simulink model "IEEE39bus"  (Simulink 8.5)
settings: Solver=ode3  SolverMode=SingleTasking  StartTime=0.0  StopTime=50  FixedStep=Ts  RelTol=1e-3
PostLoadFcn:
  | Ts=25e-6; IEEE39BusLineLength;
  | vNomHV = 345E3;fNom=50;load('Dynamicload.mat');
InitFcn:
  | Ts=25e-6; IEEE39BusLineLength;
  | vNomHV = 345E3;fNom=50;load('Dynamicload.mat');
undefined symbols (not defined in the file): D1, Delta, load15, load16, load18, load20, load21, load23, load24, load25, load26, load27, load28, load29, load3, load39, load4, load7, load8, TL_10_11_len, TL_10_13_len, TL_13_14_len, TL_14_15_len, TL_15_16_len, TL_16_17_len, TL_16_19_len, TL_16_21_len, TL_16_24_len, TL_17_18_len, TL_17_27_len, TL_1_2_len, TL_1_39_len, TL_21_22_len, TL_22_23_len, TL_24_23_len, TL_25_26_len, TL_26_27_len, TL_26_28_len, TL_26_29_len, TL_28_29_len, TL_2_25_len, TL_2_2_len, TL_3_18_len, TL_3_4_len, TL_4_14_len, TL_4_5_len, TL_5_6_len, TL_5_8_len, TL_6_11_len, TL_6_7_len, TL_7_8_len, TL_8_9_len, TL_9_39_len
libraries: powerlib x175, op_dpl_lib x34, rtlab x14, sps_avr x9, powerlib_extras x2, artemis x1, powerlib_meascontrol x1
(part 2 of 5)

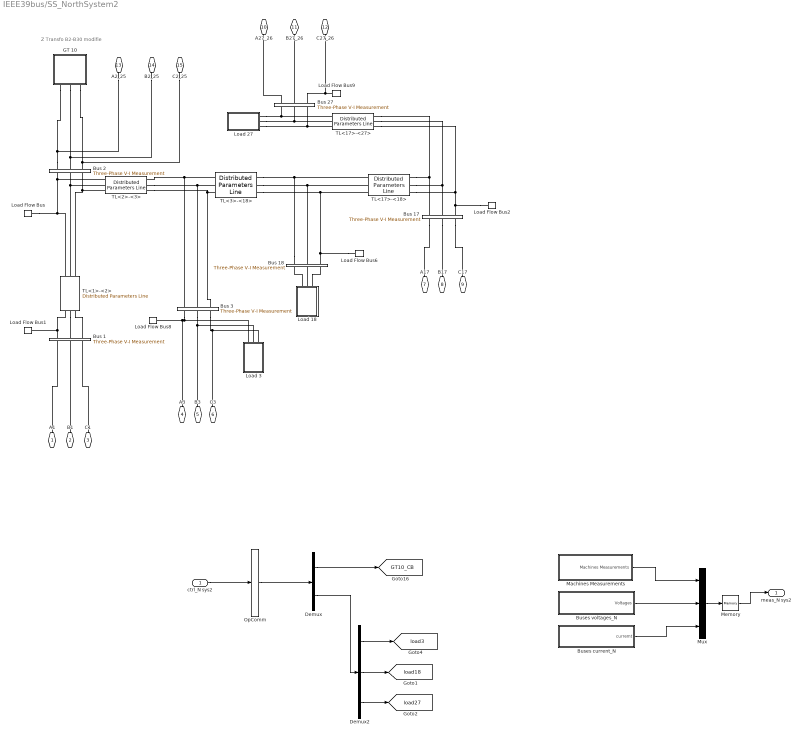
== system IEEE39bus/SS_NorthSystem2 ==
  note: Z Transfo B2-B30 modifie
  ctrl_N sys2 : Inport
  Bus 1 : powerlib/Measurements/Three-Phase V-I Measurement  VoltageMeasurement=phase-to-ground  SetLabelV=on  LabelV=V_bus_1  Vpu=off  VpuLL=off  CurrentMeasurement=yes  SetLabelI=on  LabelI=I_bus_1  Ipu=off  Pbase=100e6  Vbase=230e3  OutputType=Complex  PhasorSimulation=off  PSBequivalent=0
  Bus 17 : powerlib/Measurements/Three-Phase V-I Measurement  VoltageMeasurement=phase-to-ground  SetLabelV=on  LabelV=V_bus_17  Vpu=off  VpuLL=off  CurrentMeasurement=yes  SetLabelI=on  LabelI=I_bus_17  Ipu=off  Pbase=100e6  Vbase=230e3  OutputType=Complex  PhasorSimulation=off  PSBequivalent=0
  Bus 18 : powerlib/Measurements/Three-Phase V-I Measurement  VoltageMeasurement=phase-to-ground  SetLabelV=on  LabelV=V_bus_18  Vpu=off  VpuLL=off  CurrentMeasurement=yes  SetLabelI=on  LabelI=I_bus_18  Ipu=off  Pbase=100e6  Vbase=230e3  OutputType=Complex  PhasorSimulation=off  PSBequivalent=0
  Bus 2 : powerlib/Measurements/Three-Phase V-I Measurement  VoltageMeasurement=phase-to-ground  SetLabelV=on  LabelV=V_bus_2  Vpu=off  VpuLL=off  CurrentMeasurement=yes  SetLabelI=on  LabelI=I_bus_2  Ipu=off  Pbase=100e6  Vbase=230e3  OutputType=Complex  PhasorSimulation=off  PSBequivalent=0
  Bus 27 : powerlib/Measurements/Three-Phase V-I Measurement  VoltageMeasurement=phase-to-ground  SetLabelV=on  LabelV=V_bus_27  Vpu=off  VpuLL=off  CurrentMeasurement=yes  SetLabelI=on  LabelI=I_bus_27  Ipu=off  Pbase=100e6  Vbase=230e3  OutputType=Complex  PhasorSimulation=off  PSBequivalent=0
  Bus 3 : powerlib/Measurements/Three-Phase V-I Measurement  VoltageMeasurement=phase-to-ground  SetLabelV=on  LabelV=V_bus_3  Vpu=off  VpuLL=off  CurrentMeasurement=yes  SetLabelI=on  LabelI=I_bus_3  Ipu=off  Pbase=100e6  Vbase=230e3  OutputType=Complex  PhasorSimulation=off  PSBequivalent=0
  Buses current_N : Subsystem
  Buses voltages_N : Subsystem
  Demux : Demux  Outputs=[1 6]
  Demux2 : Demux  Outputs=[2 2 2]
  GT 10 : Subsystem
  Load 18 : Subsystem  SystemSampleTime=20e-3
  Load 27 : Subsystem  SystemSampleTime=20e-3
  Load 3 : Subsystem  SystemSampleTime=20e-3
  Load Flow Bus : powerlib/Measurements/Load Flow Bus  LConnTagsString=a  ID=Bus-2  Vbase=345e+003  Vref=1  Vangle=0  VLF=1.028  angleLF=24.05
      settings: AttributesFormatString=%<ID>\n%<Vbase>V\n%<VLF>pu\n%<angleLF>deg.
  Load Flow Bus1 : powerlib/Measurements/Load Flow Bus  LConnTagsString=a  ID=Bus-1  Vbase=345e+003  Vref=1  Vangle=0  VLF=1.036  angleLF=22.64
      settings: AttributesFormatString=%<ID>\n%<Vbase>V\n%<VLF>pu\n%<angleLF>deg.
  Load Flow Bus2 : powerlib/Measurements/Load Flow Bus  LConnTagsString=a  ID=Bus-17  Vbase=345e+003  Vref=1  Vangle=0  VLF=1.01  angleLF=19.53
      settings: AttributesFormatString=%<ID>\n%<Vbase>V\n%<VLF>pu\n%<angleLF>deg.
  Load Flow Bus6 : powerlib/Measurements/Load Flow Bus  LConnTagsString=a  ID=Bus-18  Vbase=345e+003  Vref=1  Vangle=0  VLF=1.009  angleLF=19.72
      settings: AttributesFormatString=%<ID>\n%<Vbase>V\n%<VLF>pu\n%<angleLF>deg.
  Load Flow Bus8 : powerlib/Measurements/Load Flow Bus  LConnTagsString=a  ID=Bus-3  Vbase=345e+003  Vref=1  Vangle=0  VLF=1.01  angleLF=21
      settings: AttributesFormatString=%<ID>\n%<Vbase>V\n%<VLF>pu\n%<angleLF>deg.
  Load Flow Bus9 : powerlib/Measurements/Load Flow Bus  LConnTagsString=a  ID=Bus-27  Vbase=345e+003  Vref=1  Vangle=0  VLF=1.013  angleLF=19.76
      settings: AttributesFormatString=%<ID>\n%<Vbase>V\n%<VLF>pu\n%<angleLF>deg.
  Machines Measurements : Subsystem
      mask Display: disp('Machines Measurements')
  Memory : Memory
  Mux : Mux  Inputs=3
  OpComm : rtlab/OpComm  nbport=1  groupe_acq=1  subsys_rate=0  st=0  Synchronization=on  Interpolation=on  Threshold=1.0  Missed_Data=off  Sim_Time=off  Samples=off  dynSigOut=off  from_console=0  warning_done=off  writeOpCommFile=off  Offset=off
  TL<17>-<18> : op_dpl_lib/Distributed Parameters Line  SimulationMode=ARTEMIS model  Phases=3  Frequency=50  Resistance=[0.833 3.333]/TL_17_18_len  Inductance="[0.026  0.078]/TL_17_18_len"  Capacitance=[0.294e-6 0.134e-6]/TL_17_18_len  Length=TL_17_18_len  Measurements=None
  TL<17>-<27> : op_dpl_lib/Distributed Parameters Line  SimulationMode=ARTEMIS model  Phases=3  Frequency=50  Resistance=[1.547 6.189]/TL_17_27_len  Inductance="[0.055  0.164]/TL_17_27_len"  Capacitance=[0.717e-6 0.326e-6]/TL_17_27_len  Length=TL_17_27_len  Measurements=None
  TL<1>-<2> : op_dpl_lib/Distributed Parameters Line  SimulationMode=ARTEMIS model  Phases=3  Frequency=50  Resistance=[4.166 16.66]/TL_1_2_len  Inductance="[0.13  0.389]/TL_1_2_len"  Capacitance=[1.56e-6 0.708e-6]/TL_1_2_len  Length=TL_1_2_len  Measurements=None
  TL<2>-<3> : op_dpl_lib/Distributed Parameters Line  SimulationMode=ARTEMIS model  Phases=3  Frequency=50  Resistance=[1.547 6.189]/TL_2_2_len  Inductance="[0.048  0.143]/TL_2_2_len"  Capacitance=[0.573e-6 0.261e-6]/TL_2_2_len  Length=TL_2_2_len  Measurements=None
  TL<3>-<18> : op_dpl_lib/Distributed Parameters Line  SimulationMode=ARTEMIS model  Phases=3  Frequency=50  Resistance=[1.309 5.237]/TL_3_18_len  Inductance="[0.042  0.126]/TL_3_18_len"  Capacitance=[0.476e-6 0.217e-6]/TL_3_18_len  Length=TL_3_18_len  Measurements=None
  A1 : PMIOPort  Port=1  Side=Left
  B1 : PMIOPort  Port=2  Side=Left
  C1 : PMIOPort  Port=3  Side=Left
  A3 : PMIOPort  Port=4  Side=Left
  B3 : PMIOPort  Port=5  Side=Left
  C3 : PMIOPort  Port=6  Side=Left
  A17 : PMIOPort  Port=7  Side=Left
  B17 : PMIOPort  Port=8  Side=Left
  C17 : PMIOPort  Port=9  Side=Left
  A27_26 : PMIOPort  Port=10  Side=Right
  B27_26 : PMIOPort  Port=11  Side=Right
  C27_26 : PMIOPort  Port=12  Side=Right
  A2_25 : PMIOPort  Port=13  Side=Right
  B2_25 : PMIOPort  Port=14  Side=Right
  C2_25 : PMIOPort  Port=15  Side=Right
  meas_N sys2 : Outport
  tag scope: GT10_CB=global, load18=global, load27=global, load3=global
  wires:
  Machines Measurements/1(Machines Measurements) -> Mux/1
  Mux/1 -> Memory/1
  Memory/1 -> meas_N sys2/1
  ctrl_N sys2/1 -> OpComm/1
  Buses voltages_N/1(Voltages) -> Mux/2
  Buses current_N/1(curremt) -> Mux/3
  Demux/2 -> Demux2/1
  Demux/1 -> [GT10_CB]
  Demux2/1 -> [load3]
  Demux2/3 -> [load27]
  Demux2/2 -> [load18]
  OpComm/1 -> Demux/1
  connections:
  TL<17>-<27>/LConn3 -- Load 27/LConn3 -- Bus 27/LConn3
  TL<17>-<27>/LConn2 -- Load 27/LConn2 -- Bus 27/LConn2
  TL<17>-<27>/LConn1 -- Load 27/LConn1 -- Bus 27/LConn1
  GT 10/RConn3 -- C2_25/RConn1 -- Bus 2/RConn3
  GT 10/RConn2 -- B2_25/RConn1 -- Bus 2/RConn2
  Bus 2/RConn1 -- GT 10/RConn1 -- A2_25/RConn1
  Load 18/LConn3 -- Bus 18/LConn3
  Load 18/LConn2 -- Bus 18/LConn2
  Load 18/LConn1 -- Bus 18/LConn1
  Load Flow Bus2/LConn1 -- TL<17>-<27>/RConn3 -- TL<17>-<18>/RConn3 -- Bus 17/RConn3
  TL<17>-<18>/RConn2 -- TL<17>-<27>/RConn2 -- Bus 17/RConn2
  TL<17>-<18>/RConn1 -- TL<17>-<27>/RConn1 -- Bus 17/RConn1
  TL<1>-<2>/RConn3 -- Bus 1/RConn3
  TL<1>-<2>/RConn2 -- Bus 1/RConn2
  Load Flow Bus1/LConn1 -- Bus 1/RConn1 -- TL<1>-<2>/RConn1
  TL<2>-<3>/LConn3 -- TL<1>-<2>/LConn3 -- Bus 2/LConn3
  TL<2>-<3>/LConn1 -- TL<1>-<2>/LConn1 -- Load Flow Bus/LConn1 -- Bus 2/LConn1
  TL<3>-<18>/LConn2 -- Bus 3/RConn2 -- TL<2>-<3>/RConn2
  TL<3>-<18>/LConn1 -- Bus 3/RConn1 -- TL<2>-<3>/RConn1
  TL<3>-<18>/LConn3 -- Bus 3/RConn3 -- TL<2>-<3>/RConn3
  Bus 3/LConn3 -- C3/RConn1 -- Load 3/LConn3
  Bus 3/LConn2 -- B3/RConn1 -- Load 3/LConn2
  Load Flow Bus8/LConn1 -- Load 3/LConn1 -- Bus 3/LConn1 -- A3/RConn1
  TL<2>-<3>/LConn2 -- TL<1>-<2>/LConn2 -- Bus 2/LConn2
  B1/RConn1 -- Bus 1/LConn2
  A1/RConn1 -- Bus 1/LConn1
  C1/RConn1 -- Bus 1/LConn3
  Bus 18/RConn1 -- TL<17>-<18>/LConn1 -- TL<3>-<18>/RConn1
  Bus 18/RConn2 -- TL<17>-<18>/LConn2 -- TL<3>-<18>/RConn2
  Load Flow Bus6/LConn1 -- TL<17>-<18>/LConn3 -- TL<3>-<18>/RConn3 -- Bus 18/RConn3
  Bus 17/LConn2 -- B17/RConn1
  Bus 17/LConn3 -- C17/RConn1
  Bus 17/LConn1 -- A17/RConn1
  Bus 27/RConn2 -- B27_26/RConn1
  Load Flow Bus9/LConn1 -- Bus 27/RConn3 -- C27_26/RConn1
  Bus 27/RConn1 -- A27_26/RConn1

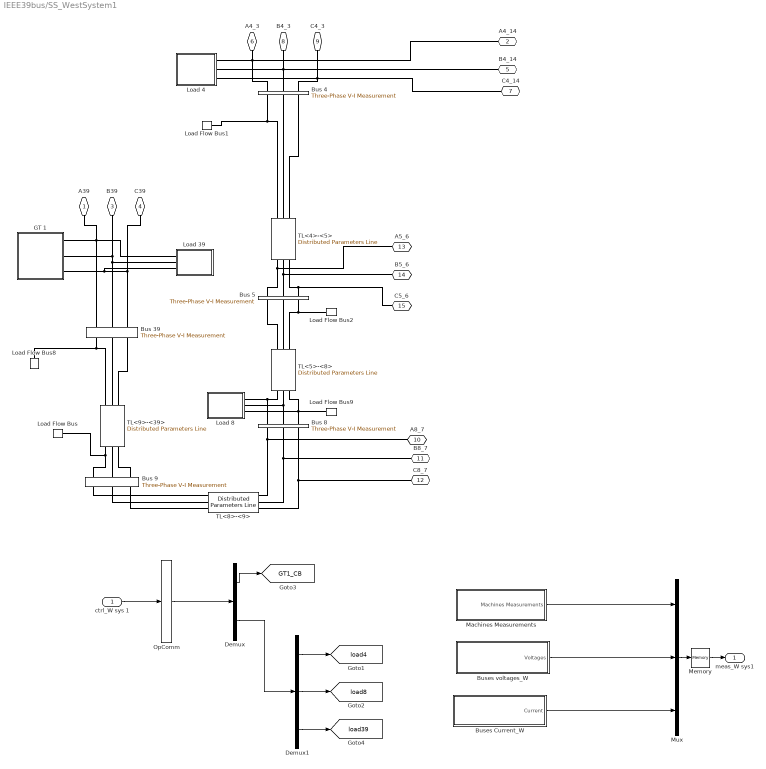
== system IEEE39bus/SS_WestSystem1 ==
  ctrl_W sys 1 : Inport
  Bus 39 : powerlib/Measurements/Three-Phase V-I Measurement  VoltageMeasurement=phase-to-ground  SetLabelV=on  LabelV=V_bus_39  Vpu=off  VpuLL=off  CurrentMeasurement=yes  SetLabelI=on  LabelI=I_bus_39  Ipu=off  Pbase=100e6  Vbase=345e3  OutputType=Complex  PhasorSimulation=off  PSBequivalent=0
  Bus 4 : powerlib/Measurements/Three-Phase V-I Measurement  VoltageMeasurement=phase-to-ground  SetLabelV=on  LabelV=V_bus_4  Vpu=off  VpuLL=off  CurrentMeasurement=yes  SetLabelI=on  LabelI=I_bus_4  Ipu=off  Pbase=100e6  Vbase=230e3  OutputType=Complex  PhasorSimulation=off  PSBequivalent=0
  Bus 5 : powerlib/Measurements/Three-Phase V-I Measurement  VoltageMeasurement=phase-to-ground  SetLabelV=on  LabelV=V_bus_5  Vpu=off  VpuLL=off  CurrentMeasurement=yes  SetLabelI=on  LabelI=I_bus_5  Ipu=off  Pbase=100e6  Vbase=230e3  OutputType=Complex  PhasorSimulation=off  PSBequivalent=0
  Bus 8 : powerlib/Measurements/Three-Phase V-I Measurement  VoltageMeasurement=phase-to-ground  SetLabelV=on  LabelV=V_bus_8  Vpu=off  VpuLL=off  CurrentMeasurement=yes  SetLabelI=on  LabelI=I_bus_8  Ipu=off  Pbase=100e6  Vbase=230e3  OutputType=Complex  PhasorSimulation=off  PSBequivalent=0
  Bus 9 : powerlib/Measurements/Three-Phase V-I Measurement  VoltageMeasurement=phase-to-ground  SetLabelV=on  LabelV=V_bus_9  Vpu=off  VpuLL=off  CurrentMeasurement=yes  SetLabelI=on  LabelI=I_bus_9  Ipu=off  Pbase=100e6  Vbase=230e3  OutputType=Complex  PhasorSimulation=off  PSBequivalent=0
  Buses Current_W : Subsystem
  Buses voltages_W : Subsystem
  Demux : Demux  Outputs=[1 6]
  Demux1 : Demux  Outputs=[2 2 2]
  "GT 1 " : Subsystem
  Load 39 : Subsystem  SystemSampleTime=20e-3
  Load 4 : Subsystem
  Load 8 : Subsystem
  Load Flow Bus : powerlib/Measurements/Load Flow Bus  LConnTagsString=a  ID=Bus-9  Vbase=345e+003  Vref=1  Vangle=0  VLF=1.022  angleLF=20.59
      settings: AttributesFormatString=%<ID>\n%<Vbase>V\n%<VLF>pu\n%<angleLF>deg.
  Load Flow Bus1 : powerlib/Measurements/Load Flow Bus  LConnTagsString=a  ID=Bus-4  Vbase=345e+003  Vref=1  Vangle=0  VLF=0.9935  angleLF=19.16
      settings: AttributesFormatString=%<ID>\n%<Vbase>V\n%<VLF>pu\n%<angleLF>deg.
  Load Flow Bus2 : powerlib/Measurements/Load Flow Bus  LConnTagsString=a  ID=Bus-5  Vbase=345e+003  Vref=1  Vangle=0  VLF=0.9982  angleLF=20.09
      settings: AttributesFormatString=%<ID>\n%<Vbase>V\n%<VLF>pu\n%<angleLF>deg.
  Load Flow Bus8 : powerlib/Measurements/Load Flow Bus  LConnTagsString=a  ID=Bus-39  Vbase=345000  Vref=1.03  Vangle=0  VLF=1.029  angleLF=21.84
      settings: AttributesFormatString=%<ID>\n%<Vbase>V\n%<VLF>pu\n%<angleLF>deg.
  Load Flow Bus9 : powerlib/Measurements/Load Flow Bus  LConnTagsString=a  ID=Bus-8  Vbase=345e+003  Vref=1  Vangle=0  VLF=0.9916  angleLF=18.81
      settings: AttributesFormatString=%<ID>\n%<Vbase>V\n%<VLF>pu\n%<angleLF>deg.
  Machines Measurements : Subsystem
      mask Display: disp('Machines Measurements')
  Memory : Memory
  Mux : Mux  Inputs=3
  OpComm : rtlab/OpComm  nbport=1  groupe_acq=1  subsys_rate=0  st=0  Synchronization=on  Interpolation=on  Threshold=1.0  Missed_Data=off  Sim_Time=off  Samples=off  dynSigOut=off  from_console=0  warning_done=off  writeOpCommFile=off  Offset=off
  TL<4>-<5> : op_dpl_lib/Distributed Parameters Line  SimulationMode=ARTEMIS model  Phases=3  Frequency=50  Resistance=[0.952 3.809]/TL_4_5_len  Inductance="[0.04  0.121]/TL_4_5_len"  Capacitance=[0.299e-6 0.136e-6]/TL_4_5_len  Length=TL_4_5_len  Measurements=None
  TL<5>-<8> : op_dpl_lib/Distributed Parameters Line  SimulationMode=ARTEMIS model  Phases=3  Frequency=50  Resistance=[0.952 3.809]/TL_5_8_len  Inductance="[0.035  0.106]/TL_5_8_len"  Capacitance=[0.329e-6 0.15e-6]/TL_5_8_len  Length=TL_5_8_len  Measurements=None
  TL<8>-<9> : op_dpl_lib/Distributed Parameters Line  SimulationMode=ARTEMIS model  Phases=3  Frequency=50  Resistance=[2.738 10.95]/TL_8_9_len  Inductance="[0.115  0.344]/TL_8_9_len"  Capacitance=[0.848e-6 0.385e-6]/TL_8_9_len  Length=TL_8_9_len  Measurements=None
  TL<9>-<39> : op_dpl_lib/Distributed Parameters Line  SimulationMode=ARTEMIS model  Phases=3  Frequency=50  Resistance=[1.19 4.761]/TL_9_39_len  Inductance="[0.079  0.237]/TL_9_39_len"  Capacitance=[2.674e-6 1.216e-6]/TL_9_39_len  Length=TL_9_39_len  Measurements=None
  A39 : PMIOPort  Port=1  Side=Right
  A4_14 : PMIOPort  Port=2  Side=Left
  B39 : PMIOPort  Port=3  Side=Right
  C39 : PMIOPort  Port=4  Side=Right
  B4_14 : PMIOPort  Port=5  Side=Left
  A4_3 : PMIOPort  Port=6  Side=Right
  C4_14 : PMIOPort  Port=7  Side=Left
  B4_3 : PMIOPort  Port=8  Side=Right
  C4_3 : PMIOPort  Port=9  Side=Right
  A8_7 : PMIOPort  Port=10  Side=Left
  B8_7 : PMIOPort  Port=11  Side=Left
  C8_7 : PMIOPort  Port=12  Side=Left
  A5_6 : PMIOPort  Port=13  Side=Right
  B5_6 : PMIOPort  Port=14  Side=Right
  C5_6 : PMIOPort  Port=15  Side=Right
  meas_W sys1 : Outport
  tag scope: GT1_CB=global, load39=global, load4=global, load8=global
  wires:
  ctrl_W sys 1/1 -> OpComm/1
  OpComm/1 -> Demux/1
  Mux/1 -> Memory/1
  Memory/1 -> meas_W sys1/1
  Buses voltages_W/1(Voltages) -> Mux/2
  Machines Measurements/1(Machines Measurements) -> Mux/1
  Buses Current_W/1(Current) -> Mux/3
  Demux/1 -> [GT1_CB]
  Demux/2 -> Demux1/1
  Demux1/2 -> [load8]
  Demux1/1 -> [load4]
  Demux1/3 -> [load39]
  connections:
  Bus 9/RConn3 -- TL<9>-<39>/RConn3
  Bus 9/RConn2 -- TL<9>-<39>/RConn2
  Bus 9/RConn1 -- Load Flow Bus/LConn1 -- TL<9>-<39>/RConn1
  Load Flow Bus9/LConn1 -- Load 8/LConn3 -- TL<5>-<8>/RConn3 -- Bus 8/RConn3
  TL<5>-<8>/RConn2 -- Load 8/LConn2 -- Bus 8/RConn2
  TL<5>-<8>/RConn1 -- Load 8/LConn1 -- Bus 8/RConn1
  TL<8>-<9>/RConn3 -- Bus 8/LConn3 -- C8_7/RConn1
  TL<8>-<9>/RConn2 -- Bus 8/LConn2 -- B8_7/RConn1
  TL<8>-<9>/RConn1 -- A8_7/RConn1 -- Bus 8/LConn1
  Bus 5/RConn3 -- TL<4>-<5>/RConn3 -- C5_6/RConn1
  Bus 5/RConn2 -- B5_6/RConn1 -- TL<4>-<5>/RConn2
  Bus 5/RConn1 -- A5_6/RConn1 -- TL<4>-<5>/RConn1
  "GT 1 "/RConn3 -- Bus 39/RConn3 -- C39/RConn1 -- Load 39/LConn3
  "GT 1 "/RConn2 -- Load 39/LConn2 -- Bus 39/RConn2 -- B39/RConn1
  Bus 39/RConn1 -- Load 39/LConn1 -- "GT 1 "/RConn1 -- A39/RConn1
  Load Flow Bus8/LConn1 -- TL<9>-<39>/LConn1 -- Bus 39/LConn1
  Bus 39/LConn2 -- TL<9>-<39>/LConn2
  Bus 39/LConn3 -- TL<9>-<39>/LConn3
  Bus 9/LConn1 -- TL<8>-<9>/LConn1
  Bus 9/LConn2 -- TL<8>-<9>/LConn2
  Bus 9/LConn3 -- TL<8>-<9>/LConn3
  Bus 5/LConn1 -- TL<5>-<8>/LConn1
  Bus 5/LConn2 -- TL<5>-<8>/LConn2
  Load Flow Bus2/LConn1 -- TL<5>-<8>/LConn3 -- Bus 5/LConn3
  Load Flow Bus1/LConn1 -- TL<4>-<5>/LConn1 -- Bus 4/LConn1
  Bus 4/LConn2 -- TL<4>-<5>/LConn2
  Bus 4/LConn3 -- TL<4>-<5>/LConn3
  B4_3/RConn1 -- B4_14/RConn1 -- Load 4/LConn2 -- Bus 4/RConn2
  A4_3/RConn1 -- A4_14/RConn1 -- Load 4/LConn1 -- Bus 4/RConn1
  C4_3/RConn1 -- C4_14/RConn1 -- Load 4/LConn3 -- Bus 4/RConn3

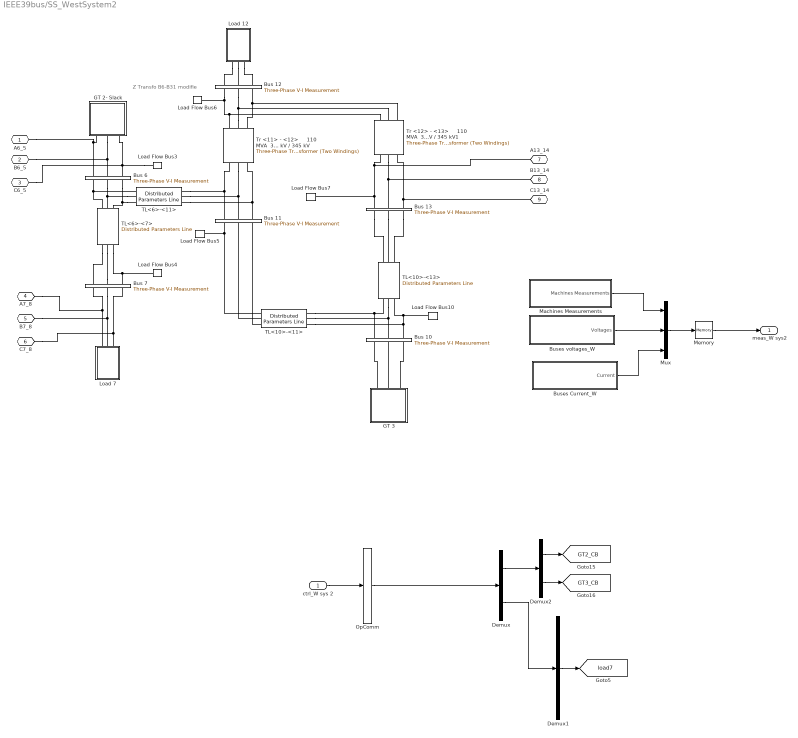
== system IEEE39bus/SS_WestSystem2 ==
  note: Z Transfo B6-B31 modifie
  ctrl_W sys 2 : Inport
  Bus 10 : powerlib/Measurements/Three-Phase V-I Measurement  VoltageMeasurement=phase-to-ground  SetLabelV=on  LabelV=V_bus_10  Vpu=off  VpuLL=off  CurrentMeasurement=yes  SetLabelI=on  LabelI=I_bus_10  Ipu=off  Pbase=100e6  Vbase=230e3  OutputType=Complex  PhasorSimulation=off  PSBequivalent=0
  Bus 11 : powerlib/Measurements/Three-Phase V-I Measurement  VoltageMeasurement=phase-to-ground  SetLabelV=on  LabelV=V_bus_11  Vpu=off  VpuLL=off  CurrentMeasurement=yes  SetLabelI=on  LabelI=I_bus_11  Ipu=off  Pbase=100e6  Vbase=230e3  OutputType=Complex  PhasorSimulation=off  PSBequivalent=0
  Bus 12 : powerlib/Measurements/Three-Phase V-I Measurement  VoltageMeasurement=phase-to-ground  SetLabelV=on  LabelV=V_bus_12  Vpu=off  VpuLL=off  CurrentMeasurement=yes  SetLabelI=on  LabelI=I_bus_12  Ipu=off  Pbase=100e6  Vbase=230e3  OutputType=Complex  PhasorSimulation=off  PSBequivalent=0
  Bus 13 : powerlib/Measurements/Three-Phase V-I Measurement  VoltageMeasurement=phase-to-ground  SetLabelV=on  LabelV=V_bus_13  Vpu=off  VpuLL=off  CurrentMeasurement=yes  SetLabelI=on  LabelI=I_bus_13  Ipu=off  Pbase=100e6  Vbase=230e3  OutputType=Complex  PhasorSimulation=off  PSBequivalent=0
  Bus 6 : powerlib/Measurements/Three-Phase V-I Measurement  VoltageMeasurement=phase-to-ground  SetLabelV=on  LabelV=V_bus_6  Vpu=off  VpuLL=off  CurrentMeasurement=yes  SetLabelI=on  LabelI=I_bus_6  Ipu=off  Pbase=100e6  Vbase=230e3  OutputType=Complex  PhasorSimulation=off  PSBequivalent=0
  Bus 7 : powerlib/Measurements/Three-Phase V-I Measurement  VoltageMeasurement=phase-to-ground  SetLabelV=on  LabelV=V_bus_7  Vpu=off  VpuLL=off  CurrentMeasurement=yes  SetLabelI=on  LabelI=I_bus_7  Ipu=off  Pbase=100e6  Vbase=230e3  OutputType=Complex  PhasorSimulation=off  PSBequivalent=0
  Buses Current_W : Subsystem
  Buses voltages_W : Subsystem
  Demux : Demux  Outputs=[2 2]
  Demux1 : Demux  Outputs=[2 ]
  Demux2 : Demux  Outputs=2
  GT 2- Slack : Subsystem
  GT 3 : Subsystem
  Load 12 : Subsystem
  Load 7 : Subsystem
  Load Flow Bus10 : powerlib/Measurements/Load Flow Bus  LConnTagsString=a  ID=Bus-10  Vbase=345e+003  Vref=1  Vangle=0  VLF=1.011  angleLF=22.22
      settings: AttributesFormatString=%<ID>\n%<Vbase>V\n%<VLF>pu\n%<angleLF>deg.
  Load Flow Bus3 : powerlib/Measurements/Load Flow Bus  LConnTagsString=a  ID=Bus-6  Vbase=345e+003  Vref=1  Vangle=0  VLF=1.003  angleLF=20.92
      settings: AttributesFormatString=%<ID>\n%<Vbase>V\n%<VLF>pu\n%<angleLF>deg.
  Load Flow Bus4 : powerlib/Measurements/Load Flow Bus  LConnTagsString=a  ID=Bus-7  Vbase=345e+003  Vref=1  Vangle=0  VLF=0.9928  angleLF=19.19
      settings: AttributesFormatString=%<ID>\n%<Vbase>V\n%<VLF>pu\n%<angleLF>deg.
  Load Flow Bus5 : powerlib/Measurements/Load Flow Bus  LConnTagsString=a  ID=Bus-11  Vbase=345e+003  Vref=1  Vangle=0  VLF=1.007  angleLF=21.76
      settings: AttributesFormatString=%<ID>\n%<Vbase>V\n%<VLF>pu\n%<angleLF>deg.
  Load Flow Bus6 : powerlib/Measurements/Load Flow Bus  LConnTagsString=a  ID=Bus-12  Vbase=345e+003  Vref=1  Vangle=0  VLF=0.996  angleLF=51.6
      settings: AttributesFormatString=%<ID>\n%<Vbase>V\n%<VLF>pu\n%<angleLF>deg.
  Load Flow Bus7 : powerlib/Measurements/Load Flow Bus  LConnTagsString=a  ID=Bus-13  Vbase=345e+003  Vref=1  Vangle=0  VLF=1.007  angleLF=21.59
      settings: AttributesFormatString=%<ID>\n%<Vbase>V\n%<VLF>pu\n%<angleLF>deg.
  Machines Measurements : Subsystem
      mask Display: disp('Machines Measurements')
  Memory : Memory
  Mux : Mux  Inputs=3
  OpComm : rtlab/OpComm  nbport=1  groupe_acq=1  subsys_rate=0  st=0  Synchronization=on  Interpolation=on  Threshold=1.0  Missed_Data=off  Sim_Time=off  Samples=off  dynSigOut=off  from_console=0  warning_done=off  writeOpCommFile=off  Offset=off
  TL<10>-<11> : op_dpl_lib/Distributed Parameters Line  SimulationMode=ARTEMIS model  Phases=3  Frequency=50  Resistance=[0.476 1.904]/TL_10_11_len  Inductance="[0.014  0.04]/TL_10_11_len"  Capacitance=[0.162e-6 0.074e-6]/TL_10_11_len  Length=TL_10_11_len  Measurements=None
  TL<10>-<13> : op_dpl_lib/Distributed Parameters Line  SimulationMode=ARTEMIS model  Phases=3  Frequency=50  Resistance=[0.476 1.904]/TL_10_13_len  Inductance="[0.014  0.04]/TL_10_13_len"  Capacitance=[0.162e-6 0.074e-6]/TL_10_13_len  Length=TL_10_13_len  Measurements=None
  TL<6>-<11> : op_dpl_lib/Distributed Parameters Line  SimulationMode=ARTEMIS model  Phases=3  Frequency=50  Resistance=[0.833 3.333]/TL_6_11_len  Inductance="[0.026  0.078]/TL_6_11_len"  Capacitance=[0.31e-6 0.141e-6]/TL_6_11_len  Length=TL_6_11_len  Measurements=None
  TL<6>-<7> : op_dpl_lib/Distributed Parameters Line  SimulationMode=ARTEMIS model  Phases=3  Frequency=50  Resistance=[0.714 2.857]/TL_6_7_len  Inductance="[0.029  0.087]/TL_6_7_len"  Capacitance=[0.252e-6 0.114e-6]/TL_6_7_len  Length=TL_6_7_len  Measurements=None
  Tr <11> - <12>     110 MVA  345 kV / 345 kV : powerlib/Elements/Three-Phase Transformer (Two Windings)  Winding1Connection=Delta (D1)  Winding2Connection=Yg  CoreType=Three single-phase transformers  SetSaturation=off  Hysteresis=off  DataFile='hysteresis'  SetInitialFlux=off  Measurements=None  UNITS=pu  NominalPower=[ 110e6 50]  Winding1="[345e3 0.0016*110/100/2   0.0435*110/100/2]"  Winding2="[ 1.006*345e3 0.0016*110/100/2   0.0435*110/100/2]"  Rm=500  Lm=500  L0=0.5  Saturation="[ 0,0  ;  0.005,1.2  ;  1.0,1.4 ]"  InitialFluxes=[ 0.8 , -0.8 , 0.7 ]  MoreParameters=off  BreakLoop=off  DataType=off  TransfoNumber=0
  Tr <12> - <13>     110 MVA  345 kV / 345 kV1 : powerlib/Elements/Three-Phase Transformer (Two Windings)  Winding1Connection=Delta (D1)  Winding2Connection=Yg  CoreType=Three single-phase transformers  SetSaturation=off  Hysteresis=off  DataFile='hysteresis'  SetInitialFlux=off  Measurements=None  UNITS=pu  NominalPower=[ 110e6 50]  Winding1="[ 345e3  0.0016*110/100/2   0.0435*110/100/2]"  Winding2="[ 1.006*345e3  0.0016*110/100/2   0.0435*110/100/2]"  Rm=500  Lm=500  L0=0.5  Saturation="[ 0,0  ;  0.005,1.2  ;  1.0,1.4 ]"  InitialFluxes=[ 0.8 , -0.8 , 0.7 ]  MoreParameters=off  BreakLoop=off  DataType=off  TransfoNumber=0
  A6_5 : PMIOPort  Port=1  Side=Left
  B6_5 : PMIOPort  Port=2  Side=Left
  C6_5 : PMIOPort  Port=3  Side=Left
  A7_8 : PMIOPort  Port=4  Side=Left
  B7_8 : PMIOPort  Port=5  Side=Left
  C7_8 : PMIOPort  Port=6  Side=Left
  A13_14 : PMIOPort  Port=7  Side=Right
  B13_14 : PMIOPort  Port=8  Side=Right
  C13_14 : PMIOPort  Port=9  Side=Right
  meas_W sys2 : Outport
  tag scope: GT2_CB=global, GT3_CB=global, load7=global
  wires:
  Mux/1 -> Memory/1
  Memory/1 -> meas_W sys2/1
  Buses voltages_W/1(Voltages) -> Mux/2
  Machines Measurements/1(Machines Measurements) -> Mux/1
  Buses Current_W/1(Current) -> Mux/3
  ctrl_W sys 2/1 -> OpComm/1
  OpComm/1 -> Demux/1
  Demux/2 -> Demux1/1
  Demux/1 -> Demux2/1
  Demux2/1 -> [GT2_CB]
  Demux2/2 -> [GT3_CB]
  Demux1/1 -> [load7]
  connections:
  Bus 7/RConn3 -- TL<6>-<7>/RConn3 -- Load Flow Bus4/LConn1
  Load Flow Bus3/LConn1 -- C6_5/RConn1 -- GT 2- Slack/RConn3 -- Bus 6/RConn3
  GT 2- Slack/RConn2 -- B6_5/RConn1 -- Bus 6/RConn2
  GT 2- Slack/RConn1 -- Bus 6/RConn1 -- A6_5/RConn1
  TL<6>-<11>/LConn3 -- TL<6>-<7>/LConn3 -- Bus 6/LConn3
  TL<6>-<11>/LConn2 -- TL<6>-<7>/LConn2 -- Bus 6/LConn2
  TL<6>-<7>/LConn1 -- Bus 6/LConn1 -- TL<6>-<11>/LConn1
  Bus 13/RConn3 -- Tr <12> - <13>     110 MVA  345 kV / 345 kV1/LConn3 -- C13_14/RConn1
  Tr <12> - <13>     110 MVA  345 kV / 345 kV1/LConn2 -- Bus 13/RConn2 -- B13_14/RConn1
  Load Flow Bus7/LConn1 -- Bus 13/RConn1 -- Tr <12> - <13>     110 MVA  345 kV / 345 kV1/LConn1 -- A13_14/RConn1
  Load 12/LConn3 -- Bus 12/RConn3
  Load 12/LConn2 -- Bus 12/RConn2
  Load 12/LConn1 -- Bus 12/RConn1
  Bus 12/LConn3 -- Tr <11> - <12>     110 MVA  345 kV / 345 kV/RConn3 -- Tr <12> - <13>     110 MVA  345 kV / 345 kV1/RConn3
  Tr <11> - <12>     110 MVA  345 kV / 345 kV/RConn2 -- Bus 12/LConn2 -- Tr <12> - <13>     110 MVA  345 kV / 345 kV1/RConn2
  Load Flow Bus6/LConn1 -- Tr <12> - <13>     110 MVA  345 kV / 345 kV1/RConn1 -- Tr <11> - <12>     110 MVA  345 kV / 345 kV/RConn1 -- Bus 12/LConn1
  Bus 11/RConn3 -- TL<6>-<11>/RConn3 -- Tr <11> - <12>     110 MVA  345 kV / 345 kV/LConn3
  Tr <11> - <12>     110 MVA  345 kV / 345 kV/LConn2 -- TL<6>-<11>/RConn2 -- Bus 11/RConn2
  Tr <11> - <12>     110 MVA  345 kV / 345 kV/LConn1 -- TL<6>-<11>/RConn1 -- Bus 11/RConn1
  TL<10>-<11>/LConn3 -- Bus 11/LConn3
  TL<10>-<11>/LConn2 -- Bus 11/LConn2
  Load Flow Bus5/LConn1 -- TL<10>-<11>/LConn1 -- Bus 11/LConn1
  TL<10>-<13>/RConn3 -- TL<10>-<11>/RConn3 -- Bus 10/RConn3 -- Load Flow Bus10/LConn1
  TL<10>-<13>/RConn2 -- TL<10>-<11>/RConn2 -- Bus 10/RConn2
  Bus 10/RConn1 -- TL<10>-<11>/RConn1 -- TL<10>-<13>/RConn1
  GT 3/RConn3 -- Bus 10/LConn3
  GT 3/RConn2 -- Bus 10/LConn2
  GT 3/RConn1 -- Bus 10/LConn1
  Bus 7/LConn1 -- A7_8/RConn1 -- Load 7/LConn1
  Bus 7/LConn2 -- Load 7/LConn2 -- B7_8/RConn1
  Bus 7/LConn3 -- C7_8/RConn1 -- Load 7/LConn3
  TL<6>-<7>/RConn2 -- Bus 7/RConn2
  TL<6>-<7>/RConn1 -- Bus 7/RConn1
  Bus 13/LConn1 -- TL<10>-<13>/LConn1
  Bus 13/LConn2 -- TL<10>-<13>/LConn2
  Bus 13/LConn3 -- TL<10>-<13>/LConn3

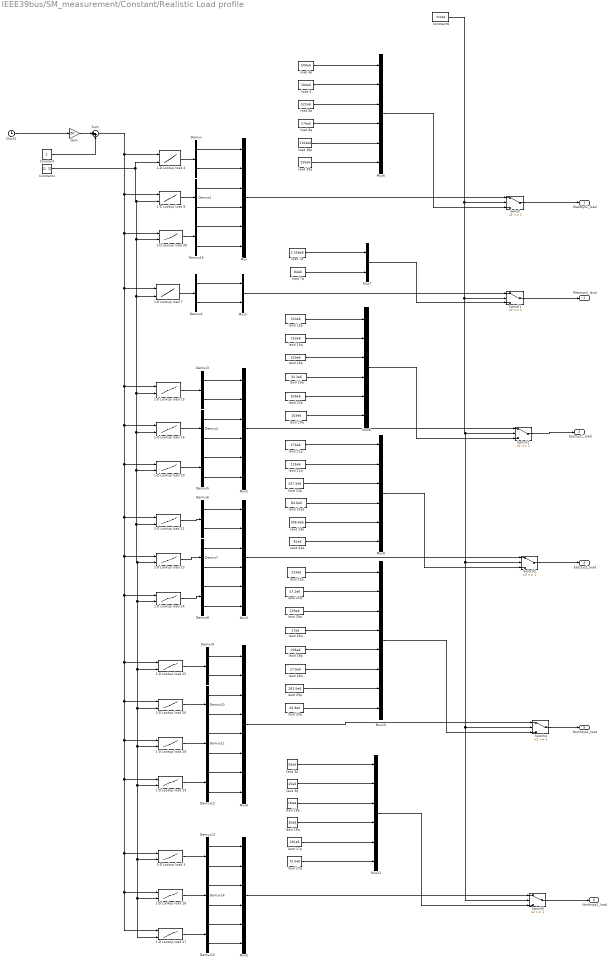
== system IEEE39bus/SM_measurement/Constant/Realistic Load profile ==
  1-D Lookup load 15 : Lookup_n-D  BreakpointsForDimension1=[1:18000]  BreakpointsForDimension2=[1 2]  Table=load15  InterpMethod=Flat  ExtrapMethod=Cubic spline  DiagnosticForOutOfRangeInput=Error  InternalRulePriority=Speed  RndMeth=Simplest  InputSameDT=on
  1-D Lookup load 16 : Lookup_n-D  BreakpointsForDimension1=[1:18000]  BreakpointsForDimension2=[1 2]  Table=load16  InterpMethod=Flat  ExtrapMethod=Cubic spline  DiagnosticForOutOfRangeInput=Error  InternalRulePriority=Speed  RndMeth=Simplest  InputSameDT=on
  1-D Lookup load 18 : Lookup_n-D  BreakpointsForDimension1=[1:18000]  BreakpointsForDimension2=[1 2]  Table=load18  InterpMethod=Flat  ExtrapMethod=Cubic spline  DiagnosticForOutOfRangeInput=Error  InternalRulePriority=Speed  RndMeth=Simplest  InputSameDT=on
  1-D Lookup load 20 : Lookup_n-D  BreakpointsForDimension1=[1:18000]  BreakpointsForDimension2=[1 2]  Table=load20  InterpMethod=Flat  ExtrapMethod=Cubic spline  DiagnosticForOutOfRangeInput=Error  InternalRulePriority=Speed  RndMeth=Simplest  InputSameDT=on
  1-D Lookup load 21 : Lookup_n-D  BreakpointsForDimension1=[1:18000]  BreakpointsForDimension2=[1 2]  Table=load21  InterpMethod=Flat  ExtrapMethod=Cubic spline  DiagnosticForOutOfRangeInput=Error  InternalRulePriority=Speed  RndMeth=Simplest  InputSameDT=on
  1-D Lookup load 23 : Lookup_n-D  BreakpointsForDimension1=[1:18000]  BreakpointsForDimension2=[1 2]  Table=load23  InterpMethod=Flat  ExtrapMethod=Cubic spline  DiagnosticForOutOfRangeInput=Error  InternalRulePriority=Speed  RndMeth=Simplest  InputSameDT=on
  1-D Lookup load 24 : Lookup_n-D  BreakpointsForDimension1=[1:18000]  BreakpointsForDimension2=[1 2]  Table=load24  InterpMethod=Flat  ExtrapMethod=Cubic spline  DiagnosticForOutOfRangeInput=Error  InternalRulePriority=Speed  RndMeth=Simplest  InputSameDT=on
  1-D Lookup load 25 : Lookup_n-D  BreakpointsForDimension1=[1:18000]  BreakpointsForDimension2=[1 2]  Table=load25  InterpMethod=Flat  ExtrapMethod=Cubic spline  DiagnosticForOutOfRangeInput=Error  InternalRulePriority=Speed  RndMeth=Simplest  InputSameDT=on
  1-D Lookup load 26 : Lookup_n-D  BreakpointsForDimension1=[1:18000]  BreakpointsForDimension2=[1 2]  Table=load26  InterpMethod=Flat  ExtrapMethod=Cubic spline  DiagnosticForOutOfRangeInput=Error  InternalRulePriority=Speed  RndMeth=Simplest  InputSameDT=on
  1-D Lookup load 27 : Lookup_n-D  BreakpointsForDimension1=[1:18000]  BreakpointsForDimension2=[1 2]  Table=load27  InterpMethod=Flat  ExtrapMethod=Cubic spline  DiagnosticForOutOfRangeInput=Error  InternalRulePriority=Speed  RndMeth=Simplest  InputSameDT=on
  1-D Lookup load 28 : Lookup_n-D  BreakpointsForDimension1=[1:18000]  BreakpointsForDimension2=[1 2]  Table=load28  InterpMethod=Flat  ExtrapMethod=Cubic spline  DiagnosticForOutOfRangeInput=Error  InternalRulePriority=Speed  RndMeth=Simplest  InputSameDT=on
  1-D Lookup load 29 : Lookup_n-D  BreakpointsForDimension1=[1:18000]  BreakpointsForDimension2=[1 2]  Table=load29  InterpMethod=Flat  ExtrapMethod=Cubic spline  DiagnosticForOutOfRangeInput=Error  InternalRulePriority=Speed  RndMeth=Simplest  InputSameDT=on
  1-D Lookup load 3 : Lookup_n-D  BreakpointsForDimension1=[1:18000]  BreakpointsForDimension2=[1 2]  Table=load3  InterpMethod=Flat  ExtrapMethod=Cubic spline  DiagnosticForOutOfRangeInput=Error  InternalRulePriority=Speed  RndMeth=Simplest  InputSameDT=on
  1-D Lookup load 39 : Lookup_n-D  BreakpointsForDimension1=[1:18000]  BreakpointsForDimension2=[1 2]  Table=load39  InterpMethod=Flat  ExtrapMethod=Cubic spline  DiagnosticForOutOfRangeInput=Error  InternalRulePriority=Speed  RndMeth=Simplest  InputSameDT=on
  1-D Lookup load 4 : Lookup_n-D  BreakpointsForDimension1=[1:18000]  BreakpointsForDimension2=[1 2]  Table=load4  InterpMethod=Flat  ExtrapMethod=Cubic spline  DiagnosticForOutOfRangeInput=Error  InternalRulePriority=Speed  RndMeth=Simplest  InputSameDT=on
  1-D Lookup load 7 : Lookup_n-D  BreakpointsForDimension1=[1:18000]  BreakpointsForDimension2=[1 2]  Table=load7  InterpMethod=Flat  ExtrapMethod=Cubic spline  DiagnosticForOutOfRangeInput=Error  InternalRulePriority=Speed  RndMeth=Simplest  InputSameDT=on
  1-D Lookup load 8 : Lookup_n-D  BreakpointsForDimension1=[1:18000]  BreakpointsForDimension2=[1 2]  Table=load8  InterpMethod=Flat  ExtrapMethod=Cubic spline  DiagnosticForOutOfRangeInput=Error  InternalRulePriority=Speed  RndMeth=Simplest  InputSameDT=on
  Clock1 : Clock
  Constant : Constant  SampleTime=20e-3
  Constant1 : Constant  Value="[1  2]"  VectorParams1D=off  SampleTime=20e-3
  Constant6 : Constant  Value=mode
  Demux{,1..16} (17 alike) : Demux  Outputs=2
  Gain : Gain  Gain=50
  Mux{,2..3,5..6,8..9,11} (8 alike) : Mux  Inputs=6
  Mux1 : Mux  Inputs=2
  Mux10 : Mux  Inputs=8
  Mux4 : Mux  Inputs=8
  Mux7 : Mux  Inputs=2
  Sum : Sum  Inputs=|++
  Switch{,1..5} (6 alike) : Switch  Threshold=1
  laod 15p : Constant  Value=320e6  VectorParams1D=off  SampleTime=20e-3
  laod 15q : Constant  Value=153e6  VectorParams1D=off  SampleTime=20e-3
  laod 16p : Constant  Value=329e6  VectorParams1D=off  SampleTime=20e-3
  laod 16q : Constant  Value=32.3e6  VectorParams1D=off  SampleTime=20e-3
  laod 18p : Constant  Value=158e6  VectorParams1D=off  SampleTime=20e-3
  laod 18q : Constant  Value=30e6  VectorParams1D=off  SampleTime=20e-3
  laod 20p : Constant  Value=628e6  VectorParams1D=off  SampleTime=20e-3
  laod 20q : Constant  Value=103e6  VectorParams1D=off  SampleTime=20e-3
  laod 21p : Constant  Value=274e6  VectorParams1D=off  SampleTime=20e-3
  laod 21q : Constant  Value=115e6  VectorParams1D=off  SampleTime=20e-3
  laod 23p : Constant  Value=247.5e6  VectorParams1D=off  SampleTime=20e-3
  laod 23p1 : Constant  Value=84.6e6  VectorParams1D=off  SampleTime=20e-3
  laod 24p : Constant  Value=308.6e6  SampleTime=20e-3
  laod 24q : Constant  Value=-92e6  VectorParams1D=off  SampleTime=20e-3
  laod 25p : Constant  Value=224e6  VectorParams1D=off  SampleTime=20e-3
  laod 25q : Constant  Value=47.2e6  VectorParams1D=off  SampleTime=20e-3
  laod 26p : Constant  Value=139e6  VectorParams1D=off  SampleTime=20e-3
  laod 26q : Constant  Value=17e6  VectorParams1D=off  SampleTime=20e-3
  laod 27p : Constant  Value=281e6  VectorParams1D=off  SampleTime=20e-3
  laod 27q : Constant  Value=75.5e6  VectorParams1D=off  SampleTime=20e-3
  laod 28p : Constant  Value=206e6  VectorParams1D=off  SampleTime=20e-3
  laod 28q : Constant  Value=27.6e6  VectorParams1D=off  SampleTime=20e-3
  laod 29p : Constant  Value=283.5e6  VectorParams1D=off  SampleTime=20e-3
  laod 29q : Constant  Value=26.9e6  VectorParams1D=off  SampleTime=20e-3
  laod 3p : Constant  Value=50e6  VectorParams1D=off  SampleTime=20e-3
  laod 3q : Constant  Value=25e6  VectorParams1D=off  SampleTime=20e-3
  load 39p : Constant  Value=1104e6  VectorParams1D=off  SampleTime=20e-3
  load 39q : Constant  Value=250e6  VectorParams1D=off  SampleTime=20e-3
  load 4 : Constant  Value=184e6  VectorParams1D=off  SampleTime=20e-3
  load 4p : Constant  Value=500e6  VectorParams1D=off  SampleTime=20e-3
  load 7p : Constant  Value=2.338e8  VectorParams1D=off  SampleTime=20e-3
  load 7q : Constant  Value=84e6  VectorParams1D=off  SampleTime=20e-3
  load 8p : Constant  Value=522e6  VectorParams1D=off  SampleTime=20e-3
  load 8q : Constant  Value=176e6  VectorParams1D=off  SampleTime=20e-3
  Westsys1_load : Outport
  Westsys2_laod : Outport  Port=2
  Eastsys1_load : Outport  Port=3
  Eastsys2_load : Outport  Port=4
  Northsys1_load : Outport  Port=5
  Northsys2_load : Outport  Port=6
  wires:
  Mux2/1 -> Switch2/1
  Constant/1 -> Sum/2
  Mux/1 -> Switch/1
  Mux1/1 -> Switch1/1
  Mux5/1 -> Switch5/1
  1-D Lookup load 15/1 -> Demux3/1
  Demux2/2 -> Mux1/2
  Demux5/2 -> Mux2/6
  Demux7/2 -> Mux3/4
  Demux10/2 -> Mux4/4
  Sum/1 -> 1-D Lookup load 28/1, 1-D Lookup load 27/1, 1-D Lookup load 18/1, 1-D Lookup load 3/1, 1-D Lookup load 29/1, 1-D Lookup load 26/1, 1-D Lookup load 25/1, 1-D Lookup load 24/1, 1-D Lookup load 23/1, 1-D Lookup load 21/1, 1-D Lookup load 20/1, 1-D Lookup load 16/1, 1-D Lookup load 15/1, 1-D Lookup load 7/1, 1-D Lookup load 39/1, 1-D Lookup load 8/1, 1-D Lookup load 4/1
  1-D Lookup load 4/1 -> Demux/1
  Demux/1 -> Mux/1
  Demux/2 -> Mux/2
  1-D Lookup load 8/1 -> Demux1/1
  Demux1/1 -> Mux/3
  Demux1/2 -> Mux/4
  Demux16/1 -> Mux/5
  Demux16/2 -> Mux/6
  1-D Lookup load 39/1 -> Demux16/1
  1-D Lookup load 7/1 -> Demux2/1
  Demux2/1 -> Mux1/1
  Demux3/1 -> Mux2/1
  Demux3/2 -> Mux2/2
  1-D Lookup load 16/1 -> Demux4/1
  Demux4/1 -> Mux2/3
  Demux4/2 -> Mux2/4
  Demux5/1 -> Mux2/5
  1-D Lookup load 20/1 -> Demux5/1
  Demux6/2 -> Mux3/2
  Demux6/1 -> Mux3/1
  1-D Lookup load 21/1 -> Demux6/1
  Demux7/1 -> Mux3/3
  1-D Lookup load 23/1 -> Demux7/1
  1-D Lookup load 24/1 -> Demux8/1
  Demux8/1 -> Mux3/5
  Demux8/2 -> Mux3/6
  Demux9/2 -> Mux4/2
  Demux9/1 -> Mux4/1
  1-D Lookup load 25/1 -> Demux9/1
  1-D Lookup load 26/1 -> Demux10/1
  Demux10/1 -> Mux4/3
  Demux11/1 -> Mux4/5
  Demux11/2 -> Mux4/6
  1-D Lookup load 28/1 -> Demux11/1
  Demux12/1 -> Mux4/7
  Demux12/2 -> Mux4/8
  1-D Lookup load 29/1 -> Demux12/1
  1-D Lookup load 3/1 -> Demux13/1
  Demux13/1 -> Mux5/1
  Demux13/2 -> Mux5/2
  Constant1/1 -> 1-D Lookup load 7/2, 1-D Lookup load 20/2, 1-D Lookup load 27/2, 1-D Lookup load 18/2, 1-D Lookup load 3/2, 1-D Lookup load 29/2, 1-D Lookup load 28/2, 1-D Lookup load 26/2, 1-D Lookup load 25/2, 1-D Lookup load 24/2, 1-D Lookup load 23/2, 1-D Lookup load 21/2, 1-D Lookup load 16/2, 1-D Lookup load 15/2, 1-D Lookup load 39/2, 1-D Lookup load 8/2, 1-D Lookup load 4/2
  Demux14/1 -> Mux5/3
  Demux14/2 -> Mux5/4
  1-D Lookup load 18/1 -> Demux14/1
  Demux15/1 -> Mux5/5
  Demux15/2 -> Mux5/6
  1-D Lookup load 27/1 -> Demux15/1
  Clock1/1 -> Gain/1
  Gain/1 -> Sum/1
  Mux6/1 -> Switch/3
  load 4p/1 -> Mux6/1
  load 4/1 -> Mux6/2
  load 8p/1 -> Mux6/3
  load 8q/1 -> Mux6/4
  load 39p/1 -> Mux6/5
  load 39q/1 -> Mux6/6
  Constant6/1 -> Switch5/2, Switch4/2, Switch3/2, Switch2/2, Switch1/2, Switch/2
  Switch/1 -> Westsys1_load/1
  Mux7/1 -> Switch1/3
  load 7q/1 -> Mux7/2
  load 7p/1 -> Mux7/1
  Switch1/1 -> Westsys2_laod/1
  Switch2/1 -> Eastsys1_load/1
  laod 20q/1 -> Mux8/6
  laod 15p/1 -> Mux8/1
  laod 15q/1 -> Mux8/2
  laod 16p/1 -> Mux8/3
  laod 16q/1 -> Mux8/4
  laod 20p/1 -> Mux8/5
  Mux8/1 -> Switch2/3
  Switch3/1 -> Eastsys2_load/1
  Mux3/1 -> Switch3/1
  laod 23p1/1 -> Mux9/4
  laod 21q/1 -> Mux9/2
  laod 21p/1 -> Mux9/1
  laod 23p/1 -> Mux9/3
  laod 24p/1 -> Mux9/5
  laod 24q/1 -> Mux9/6
  Mux9/1 -> Switch3/3
  Mux10/1 -> Switch4/3
  laod 26q/1 -> Mux10/4
  laod 25q/1 -> Mux10/2
  laod 25p/1 -> Mux10/1
  laod 26p/1 -> Mux10/3
  laod 28p/1 -> Mux10/5
  laod 28q/1 -> Mux10/6
  laod 29p/1 -> Mux10/7
  laod 29q/1 -> Mux10/8
  Switch4/1 -> Northsys1_load/1
  Mux4/1 -> Switch4/1
  Mux11/1 -> Switch5/3
  laod 3p/1 -> Mux11/1
  laod 3q/1 -> Mux11/2
  laod 18p/1 -> Mux11/3
  laod 18q/1 -> Mux11/4
  laod 27p/1 -> Mux11/5
  laod 27q/1 -> Mux11/6
  Switch5/1 -> Northsys2_load/1

== system IEEE39bus/SM_measurement/GT control ==
  note: 10
  note: 9
  note: 8
  note: 7
  note: 6
  note: 5
  note: 4
  note: 3
  note: 2
  note: 1
  Bus Creator : BusCreator  Inputs=3
  Constant{1..6,8,10,12,14} (10 alike) : Constant
  Mux1 : Mux  Inputs=3
  Mux2 : Mux
  Mux6 : Mux  Inputs=3
  GT_CBs_ctrl : Outport
  wires:
  Constant1/1 -> Mux1/2
  Constant10/1 -> Mux1/1
  Constant12/1 -> Mux2/4
  Constant5/1 -> Mux2/3
  Constant2/1 -> Mux2/2
  Constant3/1 -> Mux2/1
  Constant4/1 -> Mux6/3
  Constant8/1 -> Mux6/2
  Constant14/1 -> Mux1/3
  Constant6/1 -> Mux6/1
  Bus Creator/1 -> GT_CBs_ctrl/1
  Mux2/1 -> Bus Creator/2  "Eastsystem GT ctrl"
  Mux6/1 -> Bus Creator/1  "Westsystem GT ctrl"
  Mux1/1 -> Bus Creator/3  "Northsystem GT ctrl"

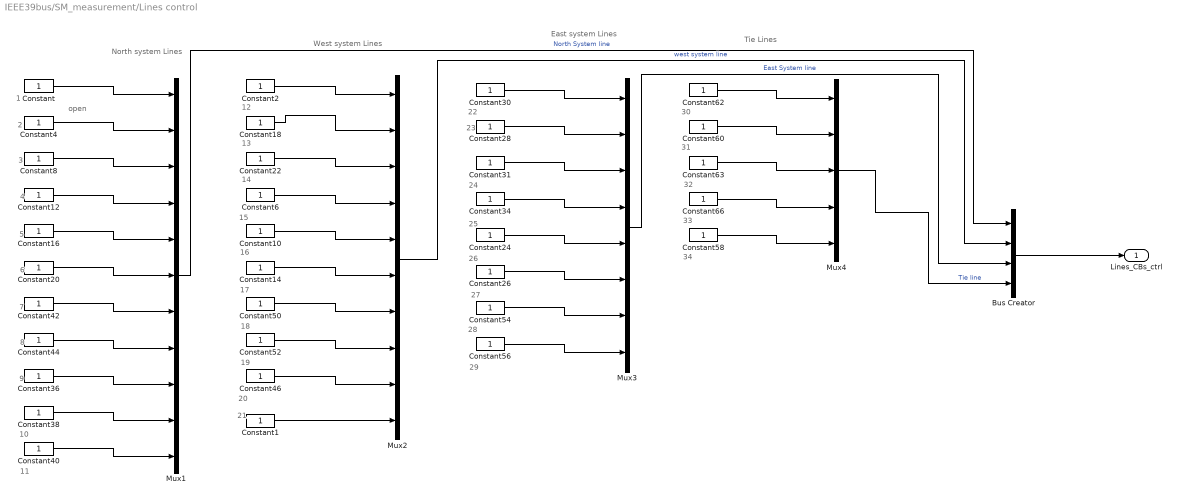
== system IEEE39bus/SM_measurement/Lines control ==
  note: 34
  note: 33
  note: 32
  note: 31
  note: 30
  note: 29
  note: 28
  note: 27
  note: 26
  note: 25
  note: 24
  note: 23
  note: 22
  note: 21
  note: 20
  note: 19
  note: 18
  note: 17
  note: 16
  note: 15
  note: 14
  note: 13
  note: 12
  note: 11
  note: 10
  note: 9
  note: 8
  note: 7
  note: 6
  note: 5
  note: 4
  note: 3
  note: 2
  note: 1
  note: open
  note: Tie Lines
  note: East system Lines
  note: West system Lines
  note: North system Lines
  Bus Creator : BusCreator
  Constant{,1..2,4,6,8,10,12,14,16,18,20,22,24,26,28,30..31,34,36,38,40,42,44,46,50,52,54,56,58,60,62..63,66} (34 alike) : Constant
  Mux1 : Mux  Inputs=11
  Mux2 : Mux  Inputs=10
  Mux3 : Mux  Inputs=8
  Mux4 : Mux  Inputs=5
  Lines_CBs_ctrl : Outport
  wires:
  Mux4/1 -> Bus Creator/4  "Tie line"
  Mux3/1 -> Bus Creator/3  "East System line"
  Mux1/1 -> Bus Creator/1  "North System line"
  Constant58/1 -> Mux4/5
  Constant66/1 -> Mux4/4
  Constant63/1 -> Mux4/3
  Constant60/1 -> Mux4/2
  Constant62/1 -> Mux4/1
  Constant56/1 -> Mux3/8
  Constant54/1 -> Mux3/7
  Constant26/1 -> Mux3/6
  Constant24/1 -> Mux3/5
  Constant34/1 -> Mux3/4
  Constant31/1 -> Mux3/3
  Constant28/1 -> Mux3/2
  Constant30/1 -> Mux3/1
  Constant1/1 -> Mux2/10
  Constant46/1 -> Mux2/9
  Constant52/1 -> Mux2/8
  Constant50/1 -> Mux2/7
  Constant14/1 -> Mux2/6
  Constant10/1 -> Mux2/5
  Constant6/1 -> Mux2/4
  Constant22/1 -> Mux2/3
  Constant18/1 -> Mux2/2
  Constant2/1 -> Mux2/1
  Constant40/1 -> Mux1/11
  Constant38/1 -> Mux1/10
  Constant36/1 -> Mux1/9
  Constant44/1 -> Mux1/8
  Constant42/1 -> Mux1/7
  Constant20/1 -> Mux1/6
  Constant16/1 -> Mux1/5
  Constant12/1 -> Mux1/4
  Constant4/1 -> Mux1/2
  Constant8/1 -> Mux1/3
  Constant/1 -> Mux1/1
  Bus Creator/1 -> Lines_CBs_ctrl/1
  Mux2/1 -> Bus Creator/2  "west system line"

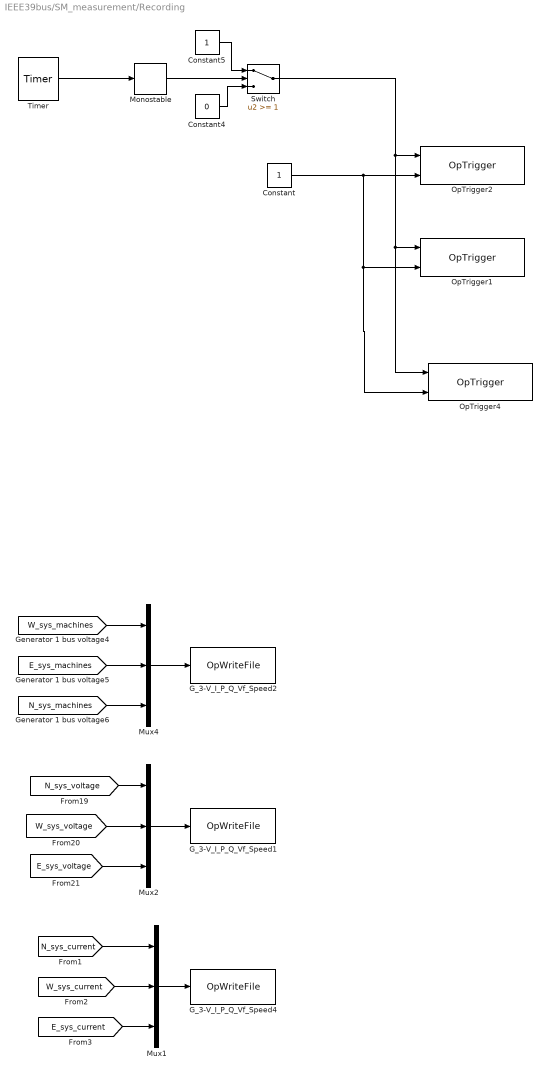
== system IEEE39bus/SM_measurement/Recording ==
  Constant : Constant
  Constant4 : Constant  Value=0
  Constant5 : Constant
  G_3-V_I_P_Q_Vf_Speed1 : rtlab/DataLogging/OpWriteFile  Static_File=on  varname=Sysvoltage  Filename=systemvoltage.mat  rtpath='./'  nrtpath='.\'  Acq_Group=28  file_size=600000000  write_offline=off  Sim_Mode=off  Nb_Samples=10000  Buffer_size=100000000
      settings: Decimation=40
  G_3-V_I_P_Q_Vf_Speed2 : rtlab/DataLogging/OpWriteFile  Static_File=on  varname=machine  Filename=machine.mat  rtpath='./'  nrtpath='.\'  Acq_Group=27  file_size=600000000  write_offline=off  Sim_Mode=off  Nb_Samples=10000  Buffer_size=100000000
      settings: Decimation=800
  G_3-V_I_P_Q_Vf_Speed4 : rtlab/DataLogging/OpWriteFile  Static_File=on  varname=Syscurrent  Filename=systemcurrrent.mat  rtpath='./'  nrtpath='.\'  Acq_Group=29  file_size=600000000  write_offline=off  Sim_Mode=off  Nb_Samples=10000  Buffer_size=100000000
      settings: Decimation=40
  Monostable : powerlib_extras/Control  Blocks/Monostable  EdgeDetect=Rising  t_mono=3700  ic=0
  Mux1 : Mux  Inputs=3
  Mux2 : Mux  Inputs=3
  Mux4 : Mux  Inputs=3
  OpTrigger1 : rtlab/DataLogging/OpTrigger  Trig_Type=TRIGGER SIGNAL >= TRIGGER LEVEL  Trig_Offset=0  Acq_Group=28
  OpTrigger2 : rtlab/DataLogging/OpTrigger  Trig_Type=TRIGGER SIGNAL >= TRIGGER LEVEL  Trig_Offset=0  Acq_Group=27
  OpTrigger4 : rtlab/DataLogging/OpTrigger  Trig_Type=TRIGGER SIGNAL >= TRIGGER LEVEL  Trig_Offset=0  Acq_Group=29
  Switch : Switch  Threshold=1
  Timer : powerlib_extras/Control  Blocks/Timer  t=[0 10 300]  e=[0 1 0 ]
  wires:
  Timer/1 -> Monostable/1
  Constant/1 -> OpTrigger2/2, OpTrigger4/2, OpTrigger1/2
  Constant4/1 -> Switch/3
  Constant5/1 -> Switch/1
  Monostable/1 -> Switch/2
  Switch/1 -> OpTrigger2/1, OpTrigger4/1, OpTrigger1/1
  Mux4/1 -> G_3-V_I_P_Q_Vf_Speed2/1
  Mux2/1 -> G_3-V_I_P_Q_Vf_Speed1/1
  [E_sys_machines] -> Mux4/2
  [W_sys_machines] -> Mux4/1
  [N_sys_voltage] -> Mux2/1
  Mux1/1 -> G_3-V_I_P_Q_Vf_Speed4/1
  [N_sys_machines] -> Mux4/3
  [W_sys_voltage] -> Mux2/2
  [E_sys_voltage] -> Mux2/3
  [N_sys_current] -> Mux1/1
  [W_sys_current] -> Mux1/2
  [E_sys_current] -> Mux1/3

== system IEEE39bus/SS_EastSystem1/Buses current_E ==
  Mux3 : Mux  Inputs=5
  current : Outport
  wires:
  Mux3/1 -> current/1
  [I_bus_14] -> Mux3/1
  [I_L15] -> Mux3/2
  [I_L16] -> Mux3/3
  [I_bus_19] -> Mux3/4
  [I_L20] -> Mux3/5

== system IEEE39bus/SS_EastSystem1/Buses voltages_E ==
  Mux3 : Mux  Inputs=5
  Voltages : Outport
  wires:
  [V_L20] -> Mux3/5
  [V_bus_19] -> Mux3/4
  [V_L16] -> Mux3/3
  [V_L15] -> Mux3/2
  [V_bus_14] -> Mux3/1
  Mux3/1 -> Voltages/1

== system IEEE39bus/SS_EastSystem1/GT 4 ==
  5 MW : powerlib/Elements/Three-Phase Parallel RLC Load  LConnTagsString=A|B|C  Configuration=Y (grounded)  NominalVoltage=22e3  NominalFrequency=50  ActivePower=5e6  InductivePower=0  CapacitivePower=0  Measurements=None  LoadType=constant Z
  Bus Selector1 : BusSelector  OutputSignals="dq0 components.Stator voltage  vq (pu),dq0 components.Stator voltage  vd (pu),Mechanical.Rotor speed  wm  (pu),Mechanical.Rotor speed deviation  dw (pu),Output active power   Peo (pu),Output reactive power  Qeo (pu)"
  Bus 33 : powerlib/Measurements/Three-Phase V-I Measurement  VoltageMeasurement=phase-to-ground  SetLabelV=on  LabelV=V_bus_G4  Vpu=off  VpuLL=off  CurrentMeasurement=no  SetLabelI=on  LabelI=I_bus_G4  Ipu=off  Pbase=100e6  Vbase=16.5e3  OutputType=Complex  PhasorSimulation=off  PSBequivalent=0
  Excitation System1 : sps_avr/Excitation System  tr=20e-3  reg=[ 200, 0.02 ]  exc=[ 1, 0 .19]  tgr=[ 0, 0 ]  damp=[ 0.0012, 1 ]  sat=[ 0, 0 ]  lim=[ 0, 7.32, 0 ]  v0=[0.9972 1.7419]
  GT1_CB4 : Subsystem
  Ground : Ground
  HTG : powerlib/Machines/Hydraulic Turbine and Governor  sm="[ 10/3  0.07 ]"  gate="[  0.01  0.97518  -0.1  0.1 ]"  reg="[  0.05  1.163  0.105  0  0.01  ]"  hyd="[  0  2.67  ]"  dref=0  po=0.57
  Load Flow Bus : powerlib/Measurements/Load Flow Bus  LConnTagsString=a  ID=Bus-33  Vbase=22000  Vref=0.9972  Vangle=0  VLF=0.9972  angleLF=-4.252
      settings: AttributesFormatString=%<ID>\n%<Vbase>V\n%<VLF>pu\n%<angleLF>deg.
  Machine 4 1000 MVA 22 kV : powerlib/Machines/Synchronous Machine pu Standard  PresetModel=No  MechanicalLoad=Mechanical power Pm  ShowDetailedParameters=on  RotorType=Round  Units=per unit standard parameters  MeasurementBus=off  NominalParameters="[ 1000E6  22000   50 ]"  Reactances1="[ 2.403 0.4 0.2 2.367 1.523 0.2 0.03  ]"  Reactances2=[ 0.995, 0.195, 0.155, 0.568, 0.143, 0.16 ]  dAxisTimeConstants=Open-circuit  qAxisTimeConstants=Open-circuit  TimeConstants1=[]  TimeConstants2=[5.69 0.03 1.5 0.04]  TimeConstants3=[]  TimeConstants4=[]  TimeConstants5=[ 9.2, 0.01, 0.01 ]  TimeConstants6=[]  TimeConstants7=[]  TimeConstants8=[]  StatorResistance=0.005  Mechanical=[ 3.117 0.02 20]  PolePairs=20  InitialConditions=[0 -47.2467 0.538718 0.538718 0.538718 -12.2371 -132.237 107.763 1.74187]  SetSaturation=off  Saturation=[0.6404,0.7127,0.8441,0.9214,0.9956,1.082,1.19,1.316,1.457;0.7,0.7698,0.8872,0.9466,0.9969,1.046,1.1,1.151,1.201]  LoadFlowParameters=[1 632000000 21938.4 0]  TsPowergui=0  TsBlock=-1  IterativeModel=Trapezoidal non iterative  BusType=PV  Pref=5.32e+008  Qref=0  Qmin=-500e6  Qmax=150e6  PLF=0  QLF=0
      settings: AttributesFormatString=\n\n
  Pref : Constant  Value=0.57
  Terminator5 : Terminator
  Transformer 4 1068.1 MVA 22 kV / 345 kV : powerlib/Elements/Three-Phase Transformer (Two Windings)  Winding1Connection=Delta (D1)  Winding2Connection=Yg  CoreType=Three single-phase transformers  SetSaturation=off  Hysteresis=off  DataFile='hysteresis'  SetInitialFlux=off  Measurements=None  UNITS=pu  NominalPower=[ 1068.1e6 50]  Winding1="[ 22e3 0.007*1068.1/100/2      0.0142*1068.1/100/2 ]"  Winding2="[ 1.07*345e3 0.007*1068.1/100/2      0.0142*1068.1/100/2]"  Rm=500  Lm=500  L0=0.5  Saturation="[ 0,0  ;  0.005,1.2  ;  1.0,1.4 ]"  InitialFluxes=[ 0.8 , -0.8 , 0.7 ]  MoreParameters=off  BreakLoop=off  DataType=off  TransfoNumber=0
  Vref : Constant  Value=0.9972
  wref : Constant
  wref4 : Constant  Value=0
  A : PMIOPort  Port=1  Side=Right
  B : PMIOPort  Port=2  Side=Right
  C : PMIOPort  Port=3  Side=Right
  tag scope: P_G4=global, Q_G4=global, V_G4=global, Wm_G4=global
  wires:
  [V_bus_G4] -> [V_G4]
  Bus Selector1/6 -> [Q_G4]  "<Output reactive power  Qeo (pu)>"
  Bus Selector1/5 -> [P_G4], HTG/4  "<Output active power   Peo (pu)>"
  Bus Selector1/4 -> HTG/5  "<Rotor speed deviation  dw (pu)>"
  Bus Selector1/3 -> [Wm_G4], HTG/3  "<Rotor speed  wm  (pu)>"
  Bus Selector1/2 -> Excitation System1/2  "<Stator voltage  vd (pu)>"
  Bus Selector1/1 -> Excitation System1/3  "<Stator voltage  vq (pu)>"
  Machine 4 1000 MVA 22 kV/1 -> Bus Selector1/1
  Excitation System1/1 -> Machine 4 1000 MVA 22 kV/2
  wref/1 -> HTG/1
  Pref/1 -> HTG/2
  Vref/1 -> Excitation System1/1
  HTG/2 -> Terminator5/1
  Ground/1 -> Excitation System1/4
  HTG/1 -> Machine 4 1000 MVA 22 kV/1
  connections:
  Machine 4 1000 MVA 22 kV/RConn3 -- Bus 33/LConn3
  Machine 4 1000 MVA 22 kV/RConn2 -- Bus 33/LConn2
  Machine 4 1000 MVA 22 kV/RConn1 -- Bus 33/LConn1
  5 MW/LConn3 -- Bus 33/RConn3 -- Transformer 4 1068.1 MVA 22 kV / 345 kV/LConn3
  5 MW/LConn2 -- Bus 33/RConn2 -- Transformer 4 1068.1 MVA 22 kV / 345 kV/LConn2
  5 MW/LConn1 -- Bus 33/RConn1 -- Load Flow Bus/LConn1 -- Transformer 4 1068.1 MVA 22 kV / 345 kV/LConn1
  GT1_CB4/LConn1 -- Transformer 4 1068.1 MVA 22 kV / 345 kV/RConn1
  GT1_CB4/LConn2 -- Transformer 4 1068.1 MVA 22 kV / 345 kV/RConn2
  GT1_CB4/LConn3 -- Transformer 4 1068.1 MVA 22 kV / 345 kV/RConn3
  C/RConn1 -- GT1_CB4/RConn3
  B/RConn1 -- GT1_CB4/RConn2
  A/RConn1 -- GT1_CB4/RConn1
